simulink model "mainSimulink"  (R2025a)
settings: Solver=FixedStepDiscrete  StartTime=0.0  StopTime=inf  FixedStep=0.001  RelTol=1e-3
undefined symbols (not defined in the file or in its folder): gray
libraries: mjLib x1
settings Model: Creator=fatur  LastModifiedBy=lkoaj104
settings SFSimCC: SimTargetLang=C++  SimDLTargetLibrary=mkl-dnn

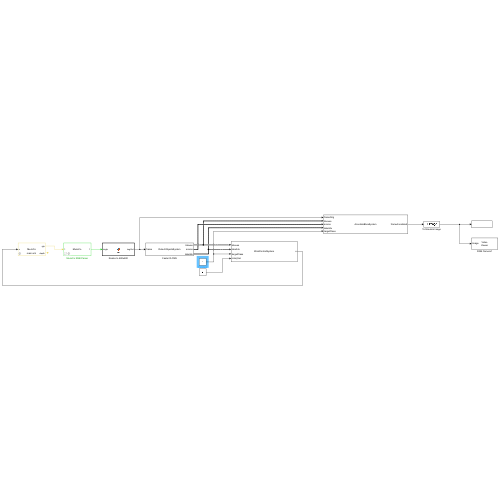
[thumbnail: Simulink's stored preview of the top-level diagram]
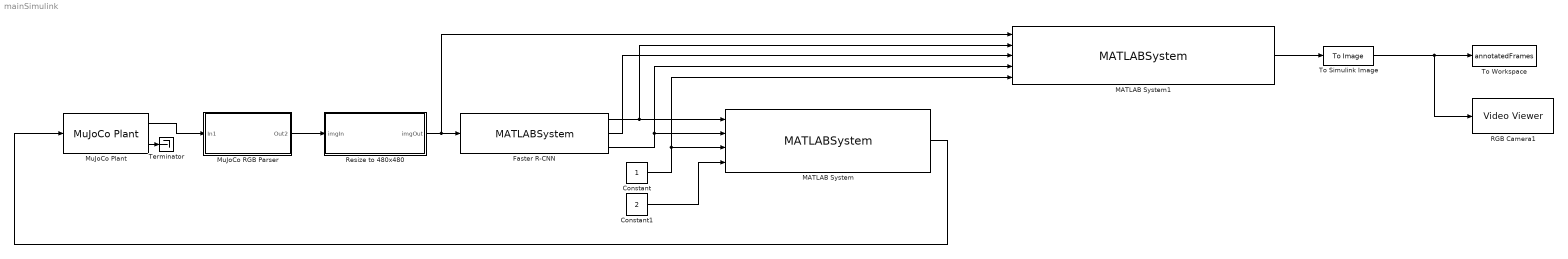
== system mainSimulink ==
  Constant : Constant
  Constant1 : Constant  Value=2
  Faster R-CNN : MATLABSystem  System=DetectObjectsSystem  ModelType=pruned_int8  ModelFolder=Model  Threshold=0.5  MaxDet=100  DetectSize=[ 480, 480 ]  SimulateUsing=Interpreted execution
      mask Type: DetectObjectsSystem
  MATLAB System : MATLABSystem  System=WindControlSystem  ExtendPos=2.5  RetractPos=0.0  MaxActiveValves=5  HoldSteps=10  RotaryVelocity=1.0  DebugMode=true  SimulateUsing=Interpreted execution
      mask Type: WindControlSystem
  MATLAB System1 : MATLABSystem  System=AnnotateBboxSystem  SimulateUsing=Interpreted execution
      mask Type: AnnotateBboxSystem
  MuJoCo Plant : mjLib/MuJoCo Plant  controlBus=[]  sensorBus=mj_bus_sensor_7979902499018342666  controlLength=[]  sensorLength=[]  rgbLength=[]  depthLength=[]  sampleTime=0.001  xmlFileRel=D:\Fatur2026\fasterRCNNClassic-Testing-Simulink\Mojoco\main.xml  xmlFile=D:\Fatur2026\fasterRCNNClassic-Testing-Simulink\Mojoco\main.xml  renderingType=Global  vsync=off  visualFPS=60  zoomLevel=1  znear=5.6517  zfar=28258.5588  cameraSampleTime=0.020  rgbOutOption=on  depthOutOption=on  controlInterfaceType=Vector
      settings: SourceProductName=MuJoCo Simulator
  MuJoCo RGB Parser : Subsystem  AncestorBlock=mjLib/MuJoCo RGB Parser  mask{inputBusType=mj_bus_rgb_3624495926710663437, selectedCamera=camera, imageRows=480, imageCols=640, startingIndex=921601, endingIndex=1843200}
      mask prompts: inputBusType "Input Type"; selectedCamera "Select Camera"
      mask TypeOptions inputBusType: mj_bus_rgb_4478678753310125630 | mj_bus_rgb_4479672711821839149
      mask Callback inputBusType:
      | inputBusType = get_param(gcb, 'inputBusType');
      | 
      | inputStruct = Simulink.Bus.createMATLABStruct(inputBusType);
      | 
      | mo = Simulink.Mask.get(gcb);
      | mo.Parameters(2).TypeOptions = fieldnames(inputStruct);
      mask TypeOptions selectedCamera: PerspectiveCamera | camera
      mask Callback selectedCamera:
      | inputBusType = get_param(gcb, 'inputBusType');
      | selectedCamera = get_param(gcb, 'selectedCamera');
      | 
      | inputStruct = Simulink.Bus.createMATLABStruct(inputBusType);
      | imageSize = size(inputStruct.(selectedCamera));
      | 
      | imageRows = imageSize(1);
      | imageCols = imageSize(2);
      | 
      | set_param(gcb, 'imageRows', num2str(imageRows));
      | set_param(gcb, 'imageCols', num2str(imageCols));
      | 
      | fields = fieldnames(inputStruct);
      | [~, camIndex] = ismember(selectedCamera, fields);
      | 
      | startingIndex = 1;
      | for i=1:(camIndex-1)
      |     imageSize = size(inputStruct.(fields{i}));
      |     startingIndex = startingIndex + imageSize(1)*imageSize(2)*imageSize(3);
      | end
      | endingIndex = startingIndex+imageSize(1) * imageSize(2)*imageSize(3) - 1;
      | 
      | set_param(gcb, 'startingIndex', num2str(startingIndex));
      | set_param(gcb, 'endingIndex', num2str(endingIndex));
      mask DialogControl Control2 Prompt: Refresh
      mask DialogControl Control2 Callback:
      | mo = Simulink.Mask.get(gcb);
      | mo.Parameters(1).TypeOptions = evalin('base', "who('mj_bus_rgb*')");
      mask Display:
      | color('black')
      | text(0.5, 0.5, 'MuJoCo', 'horizontalAlignment', 'center')
  RGB Camera1 : VideoViewer  colormapValue=gray(256)  FigPos=[966 887 904 621]
  Resize to 480x480 : MATLAB Function  TreatAsAtomicUnit=on
  Terminator : Terminator
  To Simulink Image : ToImage
  To Workspace : ToWorkspace  VariableName=annotatedFrames  SampleTime=-1
  wires:
  MuJoCo Plant/1 -> MuJoCo RGB Parser/1(In1)
  MuJoCo RGB Parser/1(Out2) -> Resize to 480x480/1(imgIn)
  To Simulink Image/1 -> To Workspace/1, RGB Camera1/1
  MATLAB System/1 -> MuJoCo Plant/1
  Faster R-CNN/1 -> MATLAB System1/2, MATLAB System/1
  Faster R-CNN/3 -> MATLAB System/2, MATLAB System1/4
  Faster R-CNN/2 -> MATLAB System1/3
  Constant/1 -> MATLAB System1/5, MATLAB System/3
  Constant1/1 -> MATLAB System/4
  MATLAB System1/1 -> To Simulink Image/1
  Resize to 480x480/1(imgOut) -> MATLAB System1/1, Faster R-CNN/1
  MuJoCo Plant/2 -> Terminator/1

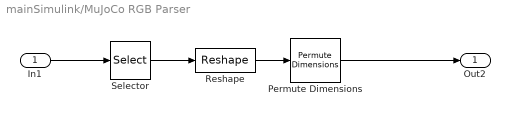
== system mainSimulink/MuJoCo RGB Parser ==
  In1 : Inport  OutDataTypeStr=uint8
  Permute Dimensions : PermuteDimensions  Order=[3 2 1]
  Reshape : Reshape  OutputDimensionality=Customize  OutputDimensions=[3,imageCols, imageRows]
  Selector : Selector  IndexOptions=Index vector (dialog)  Indices=startingIndex:endingIndex  OutputSizes=1
  Out2 : Outport
  wires:
  Selector/1 -> Reshape/1
  Reshape/1 -> Permute Dimensions/1
  In1/1 -> Selector/1
  Permute Dimensions/1 -> Out2/1

== matlab function mainSimulink/Resize to 480x480 ==
  data: imgIn input; imgOut output
function imgOut = fcn(imgIn)
%#codegen
% Letterbox resize ke 480x480 tanpa distorsi
% Input: uint8 [H x W x 3] (misal 480x640)

OUT_H = 480;
OUT_W = 480;

[inH, inW, ~] = size(imgIn);
scale = min(OUT_H / inH, OUT_W / inW);

newH = min(OUT_H, floor(inH * scale));
newW = min(OUT_W, floor(inW * scale));

padTop  = floor((OUT_H - newH) / 2);
padLeft = floor((OUT_W - newW) / 2);

imgResized = imresize(imgIn, [newH, newW]);

imgOut = zeros(OUT_H, OUT_W, 3, 'uint8');
imgOut(padTop+1 : padTop+newH, padLeft+1 : padLeft+newW, :) = imgResized;
